simulink model "Calculator"  (R2020b)
settings: configuration reference "FixedStepConfig" (kept outside this file)
settings Model: Creator=sk71149  LastModifiedBy=sk71149
settings ConfigSetRef: SourceName=FixedStepConfig  SourceLocation=Base Workspace

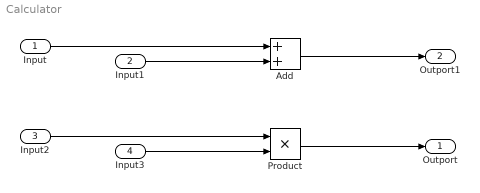
== system Calculator ==
  Input : Inport
  Input1 : Inport  Port=2
  Input2 : Inport  Port=3
  Input3 : Inport  Port=4
  Add : Sum
  Product : Product
  Outport : Outport
  Outport1 : Outport  Port=2
  wires:
  Input/1 -> Add/1
  Input1/1 -> Add/2
  Input2/1 -> Product/1
  Input3/1 -> Product/2
  Product/1 -> Outport/1
  Add/1 -> Outport1/1
